simulink model "traffic_light_stm32"  (R2014a)
settings: Solver=FixedStepDiscrete  StartTime=0.0  StopTime=10.0  FixedStep=0.1  RelTol=1e-3
model workspace (MAT data in the model file):
  Te = 0.1
libraries: simulink x5, GPIO_Lib x4
settings Model: Creator=reynaudp  LastModifiedBy=ningd
settings OptimizationCC: ExpressionDepthLimit=2147483647  OptimizeModelRefInitCode=on  LifeSpan=1
settings DebuggingCC: UnderspecifiedInitializationDetection=Classic  StateNameClashWarn=warning
settings HardwareCC: ProdLargestAtomicInteger=Integer  ProdLargestAtomicFloat=Float  ProdIntDivRoundTo=Zero  ProdEndianess=LittleEndian  ProdHWDeviceType=STMicroelectronics->STM32F4xx 32-bit Cortex-M4
settings RTWCC: SystemTargetFile=stm32F4xx.tlc  TemplateMakefile=stm32F4xx.tmf  Description=stm32F4xx (Embedded Target)  GenerateReport=on  ProcessScript=stm32F4xx_make_rtw_hook  LaunchReport=on
settings CodeAppCC: IgnoreCustomStorageClasses=off  CustomSymbolStrType=$N$R$M  InternalIdentifier=Classic
settings STFCustomTargetCC: ParMdlRefBuildCompliant=on  ConcurrentExecutionCompliant=off  IncludeMdlTerminateFcn=off  GeneratePreprocessorConditionals=Use local settings  CombineOutputUpdateFcns=on  ERTCustomFileBanners=on  SupportContinuousTime=off  SupportNonInlinedSFcns=off  MATLABClassNameForMDSCustomization=Simulink.SoftwareTarget.ERTCustomization  GRTInterface=off  SystemTargetFile=stm32F4xx.tlc
settings ERTTargetCC: GenerateSampleERTMain=off  ParMdlRefBuildCompliant=on  IncludeMdlTerminateFcn=off  ERTSrcFileBannerTemplate=sourceFileTemplate.cgt  ERTHdrFileBannerTemplate=sourceFileTemplate.cgt  ERTDataSrcFileTemplate=sourceFileTemplate.cgt  ERTDataHdrFileTemplate=sourceFileTemplate.cgt  ERTCustomFileTemplate=customRoutineProcess.tlc

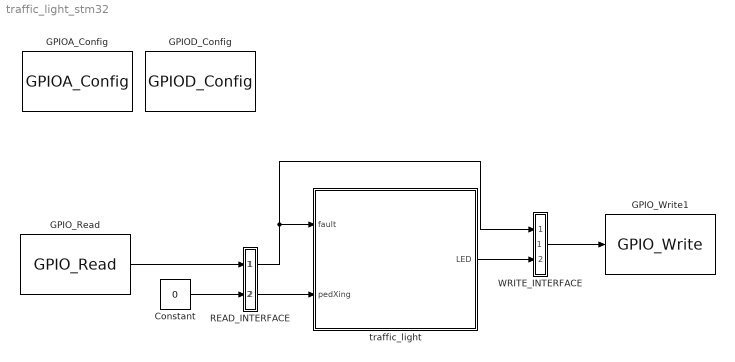
== system traffic_light_stm32 ==
  Constant : Constant  Value=0
  GPIOA_Config : GPIO_Lib/GPIOA_Config  Pin0_Use=on  Pin1_Use=off  Pin2_Use=off  Pin3_Use=off  Pin4_Use=off  Pin5_Use=off  Pin6_Use=off  Pin7_Use=off  Pin8_Use=off  Pin9_Use=off  Pin10_Use=off  Pin11_Use=off  Pin12_Use=off  Pin13_Use=off  Pin14_Use=off  Pin15_Use=off  Pin0_Speed=GPIO_Speed_50MHz  Pin1_Speed=GPIO_Speed_2MHz  Pin2_Speed=GPIO_Speed_2MHz  Pin3_Speed=GPIO_Speed_2MHz  Pin4_Speed=GPIO_Speed_2MHz  Pin5_Speed=GPIO_Speed_2MHz  Pin6_Speed=GPIO_Speed_2MHz  Pin7_Speed=GPIO_Speed_2MHz  Pin8_Speed=GPIO_Speed_2MHz  Pin9_Speed=GPIO_Speed_2MHz  Pin10_Speed=GPIO_Speed_2MHz  Pin11_Speed=GPIO_Speed_2MHz  Pin12_Speed=GPIO_Speed_2MHz  Pin13_Speed=GPIO_Speed_2MHz  Pin14_Speed=GPIO_Speed_2MHz  Pin15_Speed=GPIO_Speed_2MHz  Pin0_Mode=GPIO_Mode_IN  Pin1_Mode=GPIO_Mode_OUT  Pin2_Mode=GPIO_Mode_OUT  Pin3_Mode=GPIO_Mode_OUT  Pin4_Mode=GPIO_Mode_OUT  Pin5_Mode=GPIO_Mode_OUT  Pin6_Mode=GPIO_Mode_OUT  Pin7_Mode=GPIO_Mode_OUT  Pin8_Mode=GPIO_Mode_OUT  Pin9_Mode=GPIO_Mode_OUT  Pin10_Mode=GPIO_Mode_OUT  Pin11_Mode=GPIO_Mode_OUT  Pin12_Mode=GPIO_Mode_OUT  Pin13_Mode=GPIO_Mode_OUT  Pin14_Mode=GPIO_Mode_OUT  Pin15_Mode=GPIO_Mode_OUT  Pin0_Type=GPIO_OType_PP  Pin1_Type=GPIO_OType_PP  Pin2_Type=GPIO_OType_PP  Pin3_Type=GPIO_OType_PP  Pin4_Type=GPIO_OType_PP  Pin5_Type=GPIO_OType_PP  Pin6_Type=GPIO_OType_PP  Pin7_Type=GPIO_OType_PP  Pin8_Type=GPIO_OType_PP  Pin9_Type=GPIO_OType_PP  Pin10_Type=GPIO_OType_PP  Pin11_Type=GPIO_OType_PP  Pin12_Type=GPIO_OType_PP  Pin13_Type=GPIO_OType_PP  Pin14_Type=GPIO_OType_PP  Pin15_Type=GPIO_OType_PP  Pin0_PuPd=GPIO_PuPd_NOPULL  Pin1_PuPd=GPIO_PuPd_NOPULL  Pin2_PuPd=GPIO_PuPd_NOPULL  Pin3_PuPd=GPIO_PuPd_NOPULL  Pin4_PuPd=GPIO_PuPd_NOPULL  Pin5_PuPd=GPIO_PuPd_NOPULL  Pin6_PuPd=GPIO_PuPd_NOPULL  Pin7_PuPd=GPIO_PuPd_NOPULL  Pin8_PuPd=GPIO_PuPd_NOPULL  Pin9_PuPd=GPIO_PuPd_NOPULL  Pin10_PuPd=GPIO_PuPd_NOPULL  Pin11_PuPd=GPIO_PuPd_NOPULL  Pin12_PuPd=GPIO_PuPd_NOPULL  Pin13_PuPd=GPIO_PuPd_NOPULL  Pin14_PuPd=GPIO_PuPd_NOPULL  Pin15_PuPd=GPIO_PuPd_NOPULL  Pin0_AF=GPIO_AF_TIM2  Pin1_AF=GPIO_AF_TIM2  Pin2_AF=GPIO_AF_TIM2  Pin3_AF=GPIO_AF_TIM2  Pin4_AF=GPIO_AF_SPI1  Pin5_AF=GPIO_AF_EVENTOUT  Pin6_AF=GPIO_AF_TIM1  Pin7_AF=GPIO_AF_TIM1  Pin8_AF=GPIO_AF_MCO  Pin9_AF=GPIO_AF_TIM1  Pin10_AF=GPIO_AF_TIM1  Pin11_AF=GPIO_AF_TIM1  Pin12_AF=GPIO_AF_TIM1  Pin13_AF=GPIO_AF_SWJ  Pin14_AF=GPIO_AF_SWJ  Pin15_AF=GPIO_AF_EVENTOUT  Pin0_Set=off  Pin1_Set=off  Pin2_Set=off  Pin3_Set=off  Pin4_Set=off  Pin5_Set=off  Pin6_Set=off  Pin7_Set=off  Pin8_Set=off  Pin9_Set=off  Pin10_Set=off  Pin11_Set=off  Pin12_Set=off  Pin13_Set=off  Pin14_Set=off  Pin15_Set=off
  GPIOD_Config : GPIO_Lib/GPIOD_Config  Pin0_Use=off  Pin1_Use=off  Pin2_Use=off  Pin3_Use=off  Pin4_Use=off  Pin5_Use=off  Pin6_Use=off  Pin7_Use=off  Pin8_Use=off  Pin9_Use=off  Pin10_Use=off  Pin11_Use=off  Pin12_Use=on  Pin13_Use=on  Pin14_Use=on  Pin15_Use=on  Pin0_Speed=GPIO_Speed_2MHz  Pin1_Speed=GPIO_Speed_2MHz  Pin2_Speed=GPIO_Speed_2MHz  Pin3_Speed=GPIO_Speed_2MHz  Pin4_Speed=GPIO_Speed_2MHz  Pin5_Speed=GPIO_Speed_2MHz  Pin6_Speed=GPIO_Speed_2MHz  Pin7_Speed=GPIO_Speed_2MHz  Pin8_Speed=GPIO_Speed_2MHz  Pin9_Speed=GPIO_Speed_2MHz  Pin10_Speed=GPIO_Speed_2MHz  Pin11_Speed=GPIO_Speed_2MHz  Pin12_Speed=GPIO_Speed_50MHz  Pin13_Speed=GPIO_Speed_50MHz  Pin14_Speed=GPIO_Speed_50MHz  Pin15_Speed=GPIO_Speed_50MHz  Pin0_Mode=GPIO_Mode_OUT  Pin1_Mode=GPIO_Mode_OUT  Pin2_Mode=GPIO_Mode_OUT  Pin3_Mode=GPIO_Mode_OUT  Pin4_Mode=GPIO_Mode_OUT  Pin5_Mode=GPIO_Mode_OUT  Pin6_Mode=GPIO_Mode_OUT  Pin7_Mode=GPIO_Mode_OUT  Pin8_Mode=GPIO_Mode_OUT  Pin9_Mode=GPIO_Mode_OUT  Pin10_Mode=GPIO_Mode_OUT  Pin11_Mode=GPIO_Mode_OUT  Pin12_Mode=GPIO_Mode_OUT  Pin13_Mode=GPIO_Mode_OUT  Pin14_Mode=GPIO_Mode_OUT  Pin15_Mode=GPIO_Mode_OUT  Pin0_Type=GPIO_OType_PP  Pin1_Type=GPIO_OType_PP  Pin2_Type=GPIO_OType_PP  Pin3_Type=GPIO_OType_PP  Pin4_Type=GPIO_OType_PP  Pin5_Type=GPIO_OType_PP  Pin6_Type=GPIO_OType_PP  Pin7_Type=GPIO_OType_PP  Pin8_Type=GPIO_OType_PP  Pin9_Type=GPIO_OType_PP  Pin10_Type=GPIO_OType_PP  Pin11_Type=GPIO_OType_PP  Pin12_Type=GPIO_OType_PP  Pin13_Type=GPIO_OType_PP  Pin14_Type=GPIO_OType_PP  Pin15_Type=GPIO_OType_PP  Pin0_PuPd=GPIO_PuPd_NOPULL  Pin1_PuPd=GPIO_PuPd_NOPULL  Pin2_PuPd=GPIO_PuPd_NOPULL  Pin3_PuPd=GPIO_PuPd_NOPULL  Pin4_PuPd=GPIO_PuPd_NOPULL  Pin5_PuPd=GPIO_PuPd_NOPULL  Pin6_PuPd=GPIO_PuPd_NOPULL  Pin7_PuPd=GPIO_PuPd_NOPULL  Pin8_PuPd=GPIO_PuPd_NOPULL  Pin9_PuPd=GPIO_PuPd_NOPULL  Pin10_PuPd=GPIO_PuPd_NOPULL  Pin11_PuPd=GPIO_PuPd_NOPULL  Pin12_PuPd=GPIO_PuPd_NOPULL  Pin13_PuPd=GPIO_PuPd_NOPULL  Pin14_PuPd=GPIO_PuPd_NOPULL  Pin15_PuPd=GPIO_PuPd_NOPULL  Pin0_AF=GPIO_AF_CAN1  Pin1_AF=GPIO_AF_CAN1  Pin2_AF=GPIO_AF_TIM3  Pin3_AF=GPIO_AF_USART2  Pin4_AF=GPIO_AF_USART2  Pin5_AF=GPIO_AF_EVENTOUT  Pin6_AF=GPIO_AF_USART2  Pin7_AF=GPIO_AF_USART2  Pin8_AF=GPIO_AF_USART3  Pin9_AF=GPIO_AF_USART3  Pin10_AF=GPIO_AF_USART3  Pin11_AF=GPIO_AF_USART3  Pin12_AF=GPIO_AF_TIM4  Pin13_AF=GPIO_AF_TIM4  Pin14_AF=GPIO_AF_TIM4  Pin15_AF=GPIO_AF_EVENTOUT  Pin0_Set=off  Pin1_Set=off  Pin2_Set=off  Pin3_Set=off  Pin4_Set=off  Pin5_Set=off  Pin6_Set=off  Pin7_Set=off  Pin8_Set=off  Pin9_Set=off  Pin10_Set=off  Pin11_Set=off  Pin12_Set=off  Pin13_Set=off  Pin14_Set=off  Pin15_Set=off
  GPIO_Read : GPIO_Lib/GPIO_Read  Port_name=GPIOA  Enable_sim=off
  GPIO_Write1 : GPIO_Lib/GPIO_Write  Port_name=GPIOD  Enable_input=on  Pin0=off  Toggle_Pin0=off  Pin1=off  Toggle_Pin1=off  Pin2=off  Toggle_Pin2=off  Pin3=off  Toggle_Pin3=off  Pin4=off  Toggle_Pin4=off  Pin5=off  Toggle_Pin5=off  Pin6=off  Toggle_Pin6=off  Pin7=off  Toggle_Pin7=off  Pin8=off  Toggle_Pin8=off  Pin9=off  Toggle_Pin9=off  Pin10=off  Toggle_Pin10=off  Pin11=off  Toggle_Pin11=off  Pin12=on  Toggle_Pin12=off  Pin13=on  Toggle_Pin13=off  Pin14=on  Toggle_Pin14=off  Pin15=on  Toggle_Pin15=off
  READ_INTERFACE : Subsystem
  WRITE_INTERFACE : Subsystem
  traffic_light : Subsystem
  wires:
  traffic_light/1(LED) -> WRITE_INTERFACE/2(LEDs)
  WRITE_INTERFACE/1(LEDs_on_off) -> GPIO_Write1/1
  READ_INTERFACE/1(Out1) -> traffic_light/1(fault), WRITE_INTERFACE/1(button)
  GPIO_Read/1 -> READ_INTERFACE/1(In1)
  Constant/1 -> READ_INTERFACE/2(In2)
  READ_INTERFACE/2(Out2) -> traffic_light/2(pedXing)

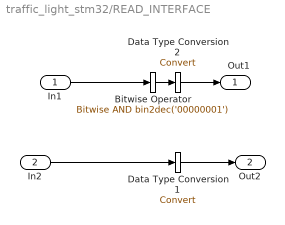
== system traffic_light_stm32/READ_INTERFACE ==
  In1 : Inport
  In2 : Inport  Port=2
  Bitwise Operator : simulink/Logic and Bit Operations/Bitwise Operator  logicop=AND  UseBitMask=on  BitMask=bin2dec('00000001')  BitMaskRealWorld=Stored Integer
  Data Type Conversion1 : DataTypeConversion
  Data Type Conversion2 : DataTypeConversion
  Out1 : Outport
  Out2 : Outport  Port=2
  wires:
  In2/1 -> Data Type Conversion1/1
  Data Type Conversion1/1 -> Out2/1
  Bitwise Operator/1 -> Data Type Conversion2/1
  Data Type Conversion2/1 -> Out1/1
  In1/1 -> Bitwise Operator/1

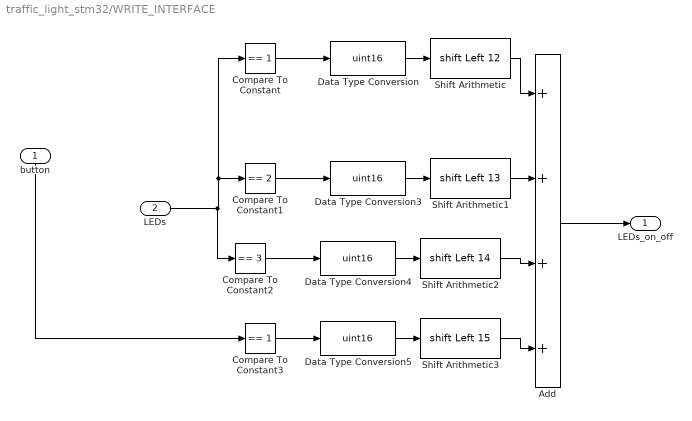
== system traffic_light_stm32/WRITE_INTERFACE ==
  button : Inport
  LEDs : Inport  Port=2
  Add : Sum  Inputs=4
  Compare To Constant : simulink/Logic and Bit Operations/Compare To Constant  relop===  const=1  OutDataTypeStr=boolean
  Compare To Constant1 : simulink/Logic and Bit Operations/Compare To Constant  relop===  const=2  OutDataTypeStr=boolean
  Compare To Constant2 : simulink/Logic and Bit Operations/Compare To Constant  relop===  const=3  OutDataTypeStr=boolean
  Compare To Constant3 : simulink/Logic and Bit Operations/Compare To Constant  relop===  const=1  OutDataTypeStr=boolean
  Data Type Conversion{,3..5} (4 alike) : DataTypeConversion  OutDataTypeStr=uint16
  Shift Arithmetic : ArithShift  BitShiftNumber=12  BitShiftDirection=Left
  Shift Arithmetic1 : ArithShift  BitShiftNumber=13  BitShiftDirection=Left
  Shift Arithmetic2 : ArithShift  BitShiftNumber=14  BitShiftDirection=Left
  Shift Arithmetic3 : ArithShift  BitShiftNumber=15  BitShiftDirection=Left
  LEDs_on_off : Outport
  wires:
  Data Type Conversion/1 -> Shift Arithmetic/1
  Compare To Constant/1 -> Data Type Conversion/1
  LEDs/1 -> Compare To Constant2/1, Compare To Constant1/1, Compare To Constant/1
  Data Type Conversion3/1 -> Shift Arithmetic1/1
  Compare To Constant3/1 -> Data Type Conversion5/1
  Shift Arithmetic3/1 -> Add/4
  Data Type Conversion5/1 -> Shift Arithmetic3/1
  Data Type Conversion4/1 -> Shift Arithmetic2/1
  Shift Arithmetic1/1 -> Add/2
  Shift Arithmetic2/1 -> Add/3
  Add/1 -> LEDs_on_off/1
  Compare To Constant1/1 -> Data Type Conversion3/1
  Compare To Constant2/1 -> Data Type Conversion4/1
  Shift Arithmetic/1 -> Add/1
  button/1 -> Compare To Constant3/1

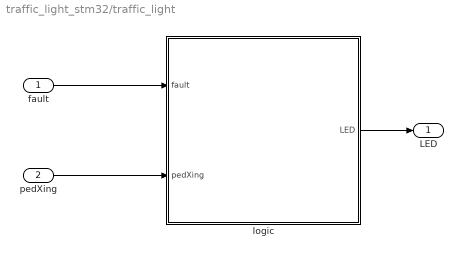
== system traffic_light_stm32/traffic_light ==
  fault : Inport
  pedXing : Inport  Port=2
  logic : Stateflow chart  TreatAsAtomicUnit=on
  LED : Outport
  wires:
  fault/1 -> logic/1(fault)
  logic/1(LED) -> LED/1
  pedXing/1 -> logic/2(pedXing)

== stateflow chart traffic_light_stm32/traffic_light/logic ==
  state Normal
    (history)
    state LIGHT_RED
      en : LED = RED;
    state LIGHT_ORANGE
      en : LED = ORANGE;
    state LIGHT_GREEN
      en : LED = GREEN;
    LIGHT_ORANGE -> LIGHT_RED : after(2/Ts,tick)
    LIGHT_RED -> LIGHT_GREEN : after(5/Ts,tick)
    LIGHT_GREEN -> LIGHT_ORANGE : [after(5/Ts,tick) | pedXing]
  state flash_LED [function]
    (default) -> (junction 44) : /* Blink */
    (junction 44) -> (junction 43) [order 1] : [LED == ORANGE]
    (junction 44) -> (junction 45) [order 2] : {LED = ORANGE;}
    (junction 43) -> (junction 42) : {LED = OFF;}
    (junction 42) -> (junction 45)
    (junction 45) -> (junction 41)
  state Faulty
    en : flash_LED()
  (default) -> LIGHT_RED
  Normal -> Faulty : [fault]
  Faulty -> Normal [order 1] : [!fault]
  Faulty -> Faulty [order 2] : after(1/Ts,tick)
  data: LED output double; OFF constant double =0; fault input; GREEN local double =1; ORANGE local double =2; RED local double =3; pedXing input uint8; Ts constant double =Te
